simulink model "PWM3"  (Simulink 7.4)
settings: Solver=ode1  SolverMode=SingleTasking  StartTime=0.0  StopTime=inf  FixedStep=0.01  MaxStep=0.02  RelTol=1e-3  AbsTol=1e-6
undefined symbols (not defined in the file or in its folder): bit
libraries: mc9s12tool x5
CloseFcn:
  | rtwprivate ssgencode ModelCloseRequest MC_AD
settings Model: Creator=fwornle  LastModifiedBy=fw  SimulationMode=external  ExtModeTrigDuration=10000
settings ConfigSet: Description=rtmc9s12target_R2009b
settings DataIOCC: LimitDataPoints=off  SaveOutput=off  SaveTime=off  SignalLoggingName=sigsOut
settings OptimizationCC: BlockReduction=off  BooleanDataType=off  InitFltsAndDblsToZero=on  OptimizeModelRefInitCode=on  LifeSpan=1
settings DebuggingCC: SaveWithParameterizedLinksMsg=none  SignalResolutionControl=TryResolveAllWithWarning  SolverPrmCheckMsg=none  MultiTaskDSMMsg=warning  MultiTaskCondExecSysMsg=none  StrictBusMsg=None
settings HardwareCC: ProdBitPerInt=16  ProdEndianess=BigEndian  ProdWordSize=16  ProdHWDeviceType=Motorola HC12
settings RTWCC: SystemTargetFile=mc9s12.tlc  GenerateMakefile=off  TemplateMakefile=mc9s12.tmf  ProcessScript=mc9s12_make_rtw_hook  IncludeERTFirstTime=on
settings CodeAppCC: IgnoreCustomStorageClasses=off
settings STFCustomTargetCC: TargetFcnLib=ansi_tfl_tmw.mat  ModelReferenceCompliant=off  IncludeMdlTerminateFcn=off  ERTCustomFileBanners=on  SupportNonInlinedSFcns=off  CPPClassGenCompliant=on  SystemTargetFile=mc9s12.tlc
settings ERTTargetCC: TargetFcnLib=ansi_tfl_tmw.mat  MultiwordLength=2048  ModelReferenceCompliant=off  ParMdlRefBuildCompliant=off  CompOptLevelCompliant=off  IncludeMdlTerminateFcn=off  CombineOutputUpdateFcns=off  ERTFirstTimeCompliant=off  SupportContinuousTime=on  ModelStepFunctionPrototypeControlCompliant=off  ExtMode=on  ExtModeMexFile=ext_serial_mc9s12_comm  ExtModeMexArgs=1,2,115200  InlinedParameterPlacement=NonHierarchical  ERTCustomFileTemplate=mc9s12_file_process.tlc  GRTInterface=on  ConvertIfToSwitch=off
settings CustomProperty: DataType=RTWOptions_EnumType_C__Users_fw__SVN_rtmc9s12-target_trunk_rtmc9s12_CW_R2009b_bin_mc9s12_1mc9s12_TargetBoard  Value=Dragon12Plus
settings EnumStrPairs: String=Dragon12

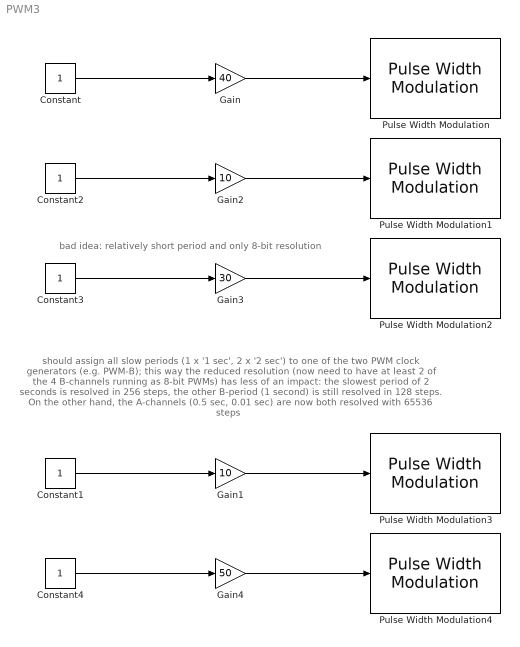
== system PWM3 ==
  note: bad idea: relatively short period and only 8-bit resolution
  note: should assign all slow periods (1 x '1 sec', 2 x '2 sec') to one of the two
      | PWM clock generators (e.g. PWM-B); this way the reduced resolution (now
      | need to have at least 2 of the 4 B-channels running as 8-bit PWMs) has less
      | of an impact: the slowest period of 2 seconds is resolved in 256 steps, the
      | other B-period (1 second) is still resolved in 128 steps. On the other hand,
      | the A-channels (0.5 sec, 0.01 sec) are now both resolved with 65536 steps
  Constant{,1..4} (5 alike) : Constant  OutDataType=sfix(16)  OutScaling=2^0
  Gain : Gain  Gain=40  ParameterDataType=sfix(16)  ParameterScaling=2^0  OutDataType=sfix(16)  OutScaling=2^0  SaturateOnIntegerOverflow=on  OutDataTypeStr=Inherit: Same as input  ParamDataTypeStr=Inherit: Same as input
  Gain1 : Gain  Gain=10  ParameterDataType=sfix(16)  ParameterScaling=2^0  OutDataType=sfix(16)  OutScaling=2^0  SaturateOnIntegerOverflow=on  OutDataTypeStr=Inherit: Same as input  ParamDataTypeStr=Inherit: Same as input
  Gain2 : Gain  Gain=10  ParameterDataType=sfix(16)  ParameterScaling=2^0  OutDataType=sfix(16)  OutScaling=2^0  SaturateOnIntegerOverflow=on  OutDataTypeStr=Inherit: Same as input  ParamDataTypeStr=Inherit: Same as input
  Gain3 : Gain  Gain=30  ParameterDataType=sfix(16)  ParameterScaling=2^0  OutDataType=sfix(16)  OutScaling=2^0  SaturateOnIntegerOverflow=on  OutDataTypeStr=Inherit: Same as input  ParamDataTypeStr=Inherit: Same as input
  Gain4 : Gain  Gain=50  ParameterDataType=sfix(16)  ParameterScaling=2^0  OutDataType=sfix(16)  OutScaling=2^0  SaturateOnIntegerOverflow=on  OutDataTypeStr=Inherit: Same as input  ParamDataTypeStr=Inherit: Same as input
  Pulse Width Modulation : mc9s12tool/Pulse Width Modulation  Tag=mcTarget_pwm  SystemSampleTime=-1  sampletime=0.01  resolution=16 bit  PWMperiod=1  pulse_pin="1  (8-bit / 16-bit)"  sign_port=PTH  sign_pin=1  Vmax=100  sig_mon=off
  Pulse Width Modulation1 : mc9s12tool/Pulse Width Modulation  Tag=mcTarget_pwm  SystemSampleTime=-1  sampletime=0.01  resolution=8 bit  PWMperiod=0.5  pulse_pin="4  (8-bit)"  sign_port=PTH  sign_pin=2  Vmax=100  sig_mon=off
  Pulse Width Modulation2 : mc9s12tool/Pulse Width Modulation  Tag=mcTarget_pwm  SystemSampleTime=-1  sampletime=0.01  resolution=8 bit  PWMperiod=0.01  pulse_pin="5  (8-bit / 16-bit)"  sign_port=PTH  sign_pin=3  Vmax=100  sig_mon=off
  Pulse Width Modulation3 : mc9s12tool/Pulse Width Modulation  Tag=mcTarget_pwm  SystemSampleTime=-1  sampletime=0.01  resolution=16 bit  PWMperiod=2  pulse_pin="3  (8-bit / 16-bit)"  sign_port=PTH  sign_pin=4  Vmax=100  sig_mon=off
  Pulse Width Modulation4 : mc9s12tool/Pulse Width Modulation  Tag=mcTarget_pwm  SystemSampleTime=-1  sampletime=0.01  resolution=16 bit  PWMperiod=2  pulse_pin="7  (8-bit / 16-bit)"  sign_port=PTH  sign_pin=5  Vmax=100  sig_mon=off
  wires:
  Gain/1 -> Pulse Width Modulation/1
  Constant/1 -> Gain/1
  Gain1/1 -> Pulse Width Modulation3/1
  Constant1/1 -> Gain1/1
  Gain2/1 -> Pulse Width Modulation1/1
  Constant2/1 -> Gain2/1
  Gain3/1 -> Pulse Width Modulation2/1
  Constant3/1 -> Gain3/1
  Gain4/1 -> Pulse Width Modulation4/1
  Constant4/1 -> Gain4/1
